simulink model "Grav_comp_final"  (R2015a)
settings: Solver=ode3  StartTime=0.0  StopTime=inf  FixedStep=1e-3  RelTol=1e-3
values from neighbouring files (symbols this model uses):
  conversion_V2mm = 17.8/(3540-260)    (= 0.00542682926829)    [Datasheet.m]    (also in setup.m)
libraries: PoliArd x6, simulink x2, dsparch4 x1
settings Model: ExtModeTrigDuration=2  Creator=User  LastModifiedBy=User
settings OptimizationCC: OptimizeModelRefInitCode=on  LifeSpan=1
settings DebuggingCC: UnderspecifiedInitializationDetection=Classic  MergeDetectMultiDrivingBlocksExec=none
settings HardwareCC: ProdLargestAtomicInteger=Long  ProdLargestAtomicFloat=Double  ProdEndianess=LittleEndian  ProdHWDeviceType=ARM Compatible->ARM Cortex
settings RTWCC: SystemTargetFile=realtime.tlc  GenerateMakefile=off  TemplateMakefile=realtime.tmf  Description=Run on Target Hardware  RTWVerbose=off
settings ERTTargetCC: CombineOutputUpdateFcns=off  ExtModeTransport=3  ExtModeMexFile=ext_serial_win32_comm_rtt  ExtModeMexArgs=0 1 9600  ERTSrcFileBannerTemplate=realtime_code_template.cgt  ERTHdrFileBannerTemplate=realtime_code_template.cgt  ERTDataSrcFileTemplate=realtime_code_template.cgt  ERTDataHdrFileTemplate=realtime_code_template.cgt  ERTCustomFileTemplate=realtime_file_process.tlc

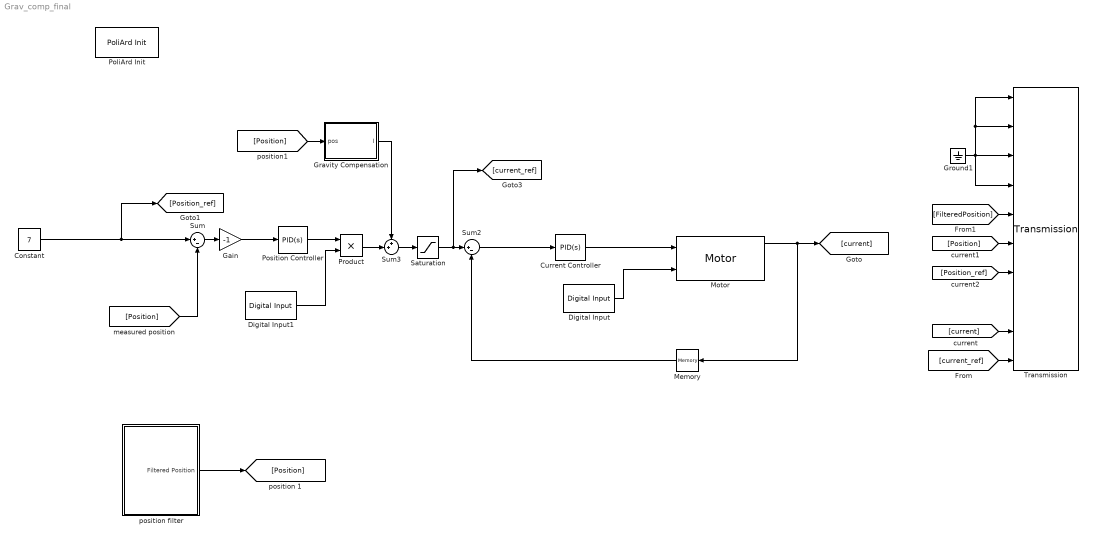
== system Grav_comp_final ==
  Constant : Constant  Value=7
  Current Controller : simulink/Continuous/PID Controller  Controller=PID  TimeDomain=Continuous-time  SampleTime=-1  IntegratorMethod=Forward Euler  FilterMethod=Forward Euler  Form=Parallel  UseFilter=on  ControllerParametersSource=internal  P=24.75  I=697  D=0  N=0  InitialConditionSource=internal  InitialConditionForIntegrator=0  InitialConditionForFilter=0  ExternalReset=none  LimitOutput=on  UpperSaturationLimit=24  LowerSaturationLimit=-24  LinearizeAsGain=on  AntiWindupMode=none  Kb=1  TrackingMode=off  Kt=1  PParamMin=[]  PParamMax=[]  IParamMin=[]  IParamMax=[]  DParamMin=[]  DParamMax=[]  NParamMin=[]  NParamMax=[]  KbParamMin=[]  KbParamMax=[]  KtParamMin=[]  KtParamMax=[]  POutMin=[]  POutMax=[]  IOutMin=[]  IOutMax=[]  DOutMin=[]  DOutMax=[]  NOutMin=[]  NOutMax=[]  KbOutMin=[]  KbOutMax=[]  KtOutMin=[]  KtOutMax=[]  IntegratorOutMin=[]  IntegratorOutMax=[]  FilterOutMin=[]  FilterOutMax=[]  SumOutMin=[]  SumOutMax=[]  SumI1OutMin=[]  SumI1OutMax=[]  SumI2OutMin=[]  SumI2OutMax=[]  SumI3OutMin=[]  SumI3OutMax=[]  SumDOutMin=[]  SumDOutMax=[]  SaturationOutMin=[]  SaturationOutMax=[]  IntegratorContinuousStateAttributes=''  IntegratorStateMustResolveToSignalObject=off  IntegratorRTWStateStorageClass=Auto  FilterContinuousStateAttributes=''  FilterStateMustResolveToSignalObject=off  FilterRTWStateStorageClass=Auto  DifferentiatorICPrevScaledInput=0  DifferentiatorOutMin=[]  DifferentiatorOutMax=[]
  Digital Input : PoliArd/Digital Input  DI_pin=3  DIsample=-1
  Digital Input1 : PoliArd/Digital Input  DI_pin=2  DIsample=-1
  Gain : Gain  Gain=-1
  Gravity Compensation : MATLAB Function  TreatAsAtomicUnit=on
  Ground1 : Ground
  Memory : Memory
  Motor : PoliArd/Motor  MotorID=2  DC_bus_mask=24  dt_mot=-1
  PoliArd Init : PoliArd/PoliArd Init
  Position Controller : simulink/Continuous/PID Controller  Controller=PID  TimeDomain=Continuous-time  SampleTime=-1  IntegratorMethod=Forward Euler  FilterMethod=Forward Euler  Form=Parallel  UseFilter=on  ControllerParametersSource=internal  P=0.07  I=0.3  D=0.01  N=100  InitialConditionSource=internal  InitialConditionForIntegrator=0  InitialConditionForFilter=0  ExternalReset=none  LimitOutput=on  UpperSaturationLimit=0.4  LowerSaturationLimit=-0.4  LinearizeAsGain=on  AntiWindupMode=back-calculation  Kb=1  TrackingMode=off  Kt=1  PParamMin=[]  PParamMax=[]  IParamMin=[]  IParamMax=[]  DParamMin=[]  DParamMax=[]  NParamMin=[]  NParamMax=[]  KbParamMin=[]  KbParamMax=[]  KtParamMin=[]  KtParamMax=[]  POutMin=[]  POutMax=[]  IOutMin=[]  IOutMax=[]  DOutMin=[]  DOutMax=[]  NOutMin=[]  NOutMax=[]  KbOutMin=[]  KbOutMax=[]  KtOutMin=[]  KtOutMax=[]  IntegratorOutMin=[]  IntegratorOutMax=[]  FilterOutMin=[]  FilterOutMax=[]  SumOutMin=[]  SumOutMax=[]  SumI1OutMin=[]  SumI1OutMax=[]  SumI2OutMin=[]  SumI2OutMax=[]  SumI3OutMin=[]  SumI3OutMax=[]  SumDOutMin=[]  SumDOutMax=[]  SaturationOutMin=[]  SaturationOutMax=[]  IntegratorContinuousStateAttributes=''  IntegratorStateMustResolveToSignalObject=off  IntegratorRTWStateStorageClass=Auto  FilterContinuousStateAttributes=''  FilterStateMustResolveToSignalObject=off  FilterRTWStateStorageClass=Auto  DifferentiatorICPrevScaledInput=0  DifferentiatorOutMin=[]  DifferentiatorOutMax=[]
  Product : Product
  Saturation : Saturate  UpperLimit=10  LowerLimit=0
  Sum : Sum  Inputs=|+-
  Sum2 : Sum  Inputs=|+-
  Sum3 : Sum  Inputs=++|
  Transmission : PoliArd/Transmission  sample_freq=100  sig_to_send=6
  position filter : Subsystem
  wires:
  Motor/1 -> Memory/1, [current]
  [Position] -> Sum/2
  Sum2/1 -> Current Controller/1
  Ground1/1 -> Transmission/4, Transmission/2, Transmission/1, Transmission/3
  Digital Input/1 -> Motor/2
  Memory/1 -> Sum2/2
  Current Controller/1 -> Motor/1
  Sum3/1 -> Saturation/1
  [Position] -> Transmission/6
  [current_ref] -> Transmission/10
  Gravity Compensation/1(I) -> Sum3/1
  Saturation/1 -> Sum2/1, [current_ref]
  Product/1 -> Sum3/2
  Position Controller/1 -> Product/1
  Digital Input1/1 -> Product/2
  Sum/1 -> Gain/1
  Gain/1 -> Position Controller/1
  Constant/1 -> [Position_ref], Sum/1
  [Position] -> Gravity Compensation/1(pos)
  [FilteredPosition] -> Transmission/5
  [current] -> Transmission/9
  [Position_ref] -> Transmission/7
  position filter/1(Filtered Position) -> [Position]

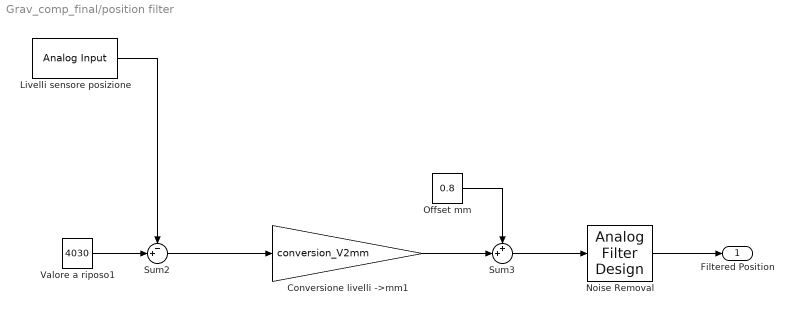
== system Grav_comp_final/position filter ==
  Conversione livelli ->mm1 : Gain  Gain=conversion_V2mm
  "Livelli sensore posizione " : PoliArd/Analog Input  AIpin_mask=2  AIsample=-1
  Noise Removal : dsparch4/Analog Filter Design  method=Butterworth  filttype=Lowpass  N=1  Wlo=150  Whi=80  Rp=2  Rs=40
  Offset mm : Constant  Value=0.8
  Sum2 : Sum  Inputs=-+|
  Sum3 : Sum  Inputs=++|
  Valore a riposo1 : Constant  Value=4030
  Filtered Position : Outport
  wires:
  "Livelli sensore posizione "/1 -> Sum2/1
  Valore a riposo1/1 -> Sum2/2
  Sum2/1 -> Conversione livelli ->mm1/1
  Conversione livelli ->mm1/1 -> Sum3/2
  Sum3/1 -> Noise Removal/1
  Offset mm/1 -> Sum3/1
  Noise Removal/1 -> Filtered Position/1

== matlab function Grav_comp_final/Gravity Compensation ==
  data: I output; pos input
function I = fcn(pos)
q=0.1115;
m = 0.1921;
I=pos*m+q;

end
